simulink model "gm_sampleModel1652_1_sub_sub"  (R2023a)
settings: Solver=VariableStepAuto  StartTime=0.0  StopTime=10.0  RelTol=1e-3
libraries: hdlsllib x7, simulink x2
settings Model: Creator=user1  LastModifiedBy=user1
settings OptimizationCC: BlockReduction=off  ConditionallyExecuteInputs=off
settings DebuggingCC: InheritedTsInSrcMsg=none

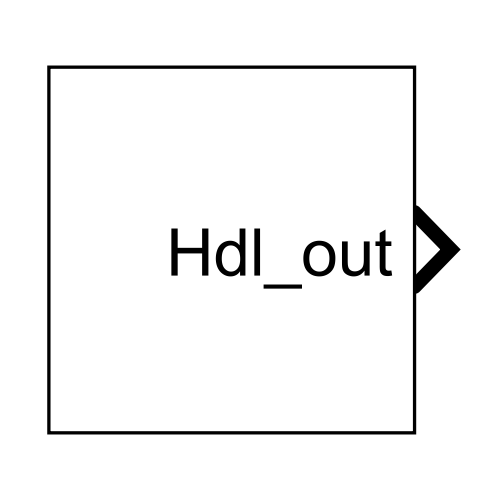
[thumbnail: Simulink's stored preview of the top-level diagram]
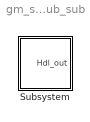
== system gm_sampleModel1652_1_sub_sub ==
  Subsystem : Subsystem

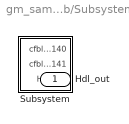
== system gm_sampleModel1652_1_sub_sub/Subsystem ==
  Subsystem : Subsystem
  Hdl_out : Outport  OutDataTypeStr=uint8

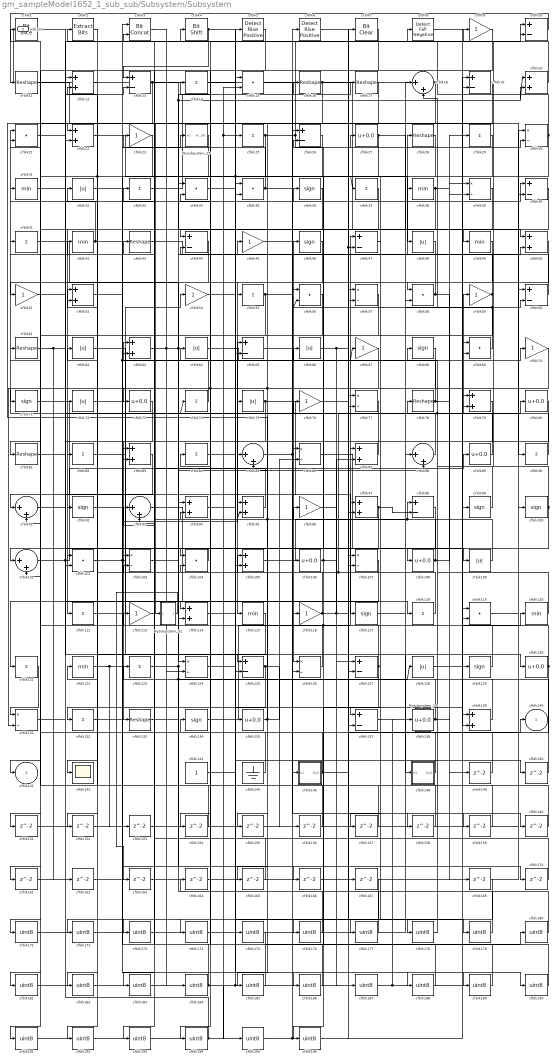
== system gm_sampleModel1652_1_sub_sub/Subsystem/Subsystem ==
  Mysubsystem_15 : Subsystem  TreatAsAtomicUnit=on  RTWFcnName=Mysubsystem_15
      settings: RTWFcnNameOpts=User specified  RTWFileNameOpts=Use function name
  Mysubsystem_19 : Subsystem  TreatAsAtomicUnit=on  RTWFcnName=Mysubsystem_19
      settings: RTWFcnNameOpts=User specified  RTWFileNameOpts=Use function name
  Mysubsystem_31 : Subsystem  TreatAsAtomicUnit=on  RTWFcnName=Mysubsystem_31
      settings: RTWFcnNameOpts=User specified  RTWFileNameOpts=Use function name
  cfblk1 : hdlsllib/Logic and Bit Operations/Bit Slice  lidx=7  ridx=0
  cfblk{10,13,19,26,40,44,47,60,65,98,125,127,137} (13 alike) : Sum  Inputs=+-  OutDataTypeStr=uint8
  cfblk{36,46,68,71,92,99..100,117,129,134} (10 alike) : Signum
  cfblk{18,85,88,91,93,101} (6 alike) : Sum  Inputs=|++  OutDataTypeStr=uint8
  cfblk{15,21,34..35,56,58,69,102,104,119} (10 alike) : DotProduct  OutDataTypeStr=uint8
  cfblk{30,39,57,77,86,103,107,124,126,131} (10 alike) : Product  Inputs=*/  OutDataTypeStr=uint8  RndMeth=Zero  SaturateOnIntegerOverflow=on
  cfblk{12,20,22,50,52,63,79,83,87,94..95,97,105,114,139} (15 alike) : Sum  OutDataTypeStr=uint8
  cfblk{27,73,80,89,106,108,130,135,138} (9 alike) : Bias  Bias=0.0  SaturateOnIntegerOverflow=off
  cfblk{32,48,62,64,66,72,75,109,128} (9 alike) : Abs  OutDataTypeStr=uint8  SaturateOnIntegerOverflow=off
  cfblk{11,16..17,28,43,61,78,81,133} (9 alike) : Reshape
  cfblk{14,25,29,33,37,41,55,74,82,84,90,112,118,121,123,132} (16 alike) : Sum  Inputs=+  OutDataTypeStr=uint8
  cfblk{9,23,45,51,54,59,67,70,76,96,113,116} (12 alike) : Gain  OutDataTypeStr=uint8
  cfblk{31,38,42,49,115,120,122} (7 alike) : MinMax  OutDataTypeStr=uint8
  cfblk142 : Scope
  cfblk144 : Constant  OutDataTypeStr=uint8  SampleTime=-1
  cfblk145 : Ground
  cfblk146 : Subsystem
      settings: LibrarySourceBlock=|
      | hdlsllib/Ports &
      | Subsystems/Subsystem
  cfblk148 : Subsystem
      settings: LibrarySourceBlock=|
      | hdlsllib/Ports &
      | Subsystems/Subsystem
  cfblk{149..167,169..170} (21 alike) : Delay  SampleTime=1
  cfblk{171..196} (26 alike) : DataTypeConversion  OutDataTypeStr=uint8  SaturateOnIntegerOverflow=off  RndMeth=Floor
  cfblk2 : simulink/Logic and Bit Operations/Extract Bits  bitsToExtract=Upper half  numBits=8  bitIdxRange=[0 7]  outScalingMode=Preserve fixed-point scaling
      settings: LibrarySourceBlock=|
      | hdlsllib/Logic and Bit
      | Operations/Extract Bits
  cfblk3 : hdlsllib/Logic and Bit Operations/Bit Concat  numInputs=2
  cfblk4 : hdlsllib/Logic and Bit Operations/Bit Shift  mode=Shift Left Logical  N=0
  cfblk5 : hdlsllib/Logic and Bit Operations/Detect Rise Positive  vinit=0  OutDataTypeStr=uint8
  cfblk6 : hdlsllib/Logic and Bit Operations/Detect Rise Positive  vinit=0  OutDataTypeStr=uint8
  cfblk7 : simulink/Logic and Bit Operations/Bit Clear  iBit=0
      settings: LibrarySourceBlock=|
      | hdlsllib/Logic and Bit
      | Operations/Bit Clear
  cfblk8 : hdlsllib/Logic and Bit Operations/Detect Fall Negative  vinit=0  OutDataTypeStr=uint8
  cfblk140 : Outport  OutDataTypeStr=uint8  VectorParamsAs1DForOutWhenUnconnected=off
  cfblk141 : Outport  Port=2  OutDataTypeStr=uint8  VectorParamsAs1DForOutWhenUnconnected=off
  Hdl_out : Outport  Port=3  OutDataTypeStr=uint8
  wires:
  cfblk125/1 -> cfblk156/1, cfblk132/1
  cfblk106/1 -> cfblk56/1, cfblk127/1
  cfblk67/1 -> cfblk155/1, cfblk131/2
  cfblk130/1 -> cfblk61/1, cfblk134/1
  cfblk72/1 -> cfblk46/1
  cfblk118/1 -> cfblk42/1, cfblk21/1
  cfblk65/1 -> cfblk126/1
  cfblk135/1 -> cfblk86/2, cfblk95/2, cfblk22/1
  cfblk78/1 -> cfblk29/1, cfblk43/1
  cfblk101/1 -> cfblk10/2, cfblk89/1
  cfblk10/1 -> cfblk11/1
  cfblk82/1 -> cfblk54/1
  cfblk99/1 -> cfblk66/1, cfblk74/1
  cfblk18/1 -> Hdl_out/1, cfblk22/2
  cfblk25/1 -> cfblk65/2, cfblk27/1, cfblk10/1
  cfblk59/1 -> cfblk28/1, cfblk56/2, cfblk127/2
  cfblk50/1 -> cfblk115/1
  cfblk29/1 -> cfblk114/1
  cfblk33/1 -> cfblk16/1
  cfblk68/1 -> cfblk112/1
  cfblk90/1 -> cfblk59/1
  cfblk95/1 -> cfblk33/1
  cfblk107/1 -> cfblk121/1
  cfblk93/1 -> cfblk146/1(In1)
  cfblk19/1 -> cfblk181/1
  cfblk40/1 -> cfblk92/1
  cfblk22/1 -> cfblk48/1
  cfblk36/1 -> cfblk44/1
  cfblk47/1 -> cfblk137/1
  cfblk73/1 -> cfblk133/1
  cfblk126/1 -> cfblk52/1
  cfblk108/1 -> cfblk39/2, cfblk65/1
  cfblk146/1(Out1) -> cfblk140/1, cfblk123/1
  cfblk109/1 -> cfblk98/1, cfblk41/1
  cfblk21/1 -> cfblk116/1
  cfblk74/1 -> cfblk63/1
  cfblk89/1 -> cfblk32/1
  cfblk144/1 -> cfblk35/2
  cfblk129/1 -> cfblk62/1
  cfblk62/1 -> cfblk148/1(In1)
  cfblk60/1 -> cfblk14/1
  cfblk134/1 -> cfblk47/1
  cfblk137/1 -> cfblk79/2
  cfblk92/1 -> cfblk108/1
  cfblk4/1 -> cfblk13/1, cfblk37/1, cfblk137/2
  cfblk38/1 -> cfblk161/1, cfblk39/1
  cfblk55/1 -> cfblk73/1, cfblk6/1
  cfblk66/1 -> cfblk167/1, cfblk69/2
  cfblk100/1 -> cfblk177/1, cfblk9/1
  cfblk43/1 -> cfblk45/1
  cfblk30/1 -> cfblk106/1, cfblk2/1
  cfblk16/1 -> cfblk90/1, cfblk125/1
  cfblk71/1 -> cfblk117/1
  cfblk63/1 -> cfblk124/2, cfblk50/2, cfblk118/1
  cfblk51/1 -> cfblk40/1
  cfblk8/1 -> cfblk129/1
  cfblk58/1 -> cfblk169/1, cfblk51/1
  cfblk119/1 -> cfblk100/1
  cfblk105/1 -> cfblk18/1
  cfblk49/1 -> cfblk58/1
  cfblk69/1 -> cfblk18/2
  cfblk112/1 -> cfblk15/1
  cfblk138/1 -> cfblk149/1, cfblk26/2
  cfblk27/1 -> cfblk49/1, cfblk83/2, cfblk105/2
  cfblk86/1 -> cfblk139/1
  cfblk102/1 -> cfblk95/1, cfblk87/1
  cfblk128/1 -> cfblk120/1
  cfblk79/1 -> cfblk83/1
  cfblk120/1 -> cfblk78/1
  cfblk42/1 -> cfblk166/1, cfblk31/1
  cfblk97/1 -> cfblk98/2, cfblk101/1
  cfblk11/1 -> cfblk60/1
  cfblk26/1 -> cfblk71/1
  cfblk1/1 -> cfblk104/1
  cfblk132/1 -> cfblk67/1, Mysubsystem_15/1(In1)
  cfblk2/1 -> cfblk82/1
  cfblk77/1 -> cfblk194/1
  cfblk12/1 -> cfblk102/1
  cfblk87/1 -> cfblk85/1
  cfblk70/1 -> cfblk154/1, cfblk114/2
  cfblk3/1 -> cfblk184/1
  cfblk46/1 -> cfblk91/1
  cfblk104/1 -> cfblk103/1
  cfblk35/1 -> cfblk139/2, cfblk23/1
  cfblk23/1 -> cfblk192/1, cfblk81/1
  cfblk20/1 -> cfblk8/1
  cfblk41/1 -> cfblk124/1
  cfblk75/1 -> cfblk93/2, cfblk107/2
  cfblk64/1 -> cfblk70/1
  cfblk121/1 -> cfblk131/1
  cfblk57/1 -> cfblk191/1
  cfblk13/1 -> cfblk172/1, cfblk50/1
  cfblk80/1 -> cfblk102/2
  cfblk148/1(Out1) -> cfblk122/1
  cfblk44/1 -> cfblk72/1
  cfblk133/1 -> cfblk128/1, cfblk17/1, cfblk20/1
  cfblk81/1 -> cfblk80/1
  cfblk122/1 -> cfblk153/1, cfblk69/1
  cfblk127/1 -> cfblk176/1, cfblk105/1, cfblk76/1
  cfblk131/1 -> cfblk13/2
  cfblk61/1 -> cfblk162/1, cfblk125/2
  cfblk116/1 -> cfblk12/2, cfblk87/2, cfblk30/2, cfblk47/2
  cfblk103/1 -> cfblk88/2
  cfblk85/1 -> cfblk160/1, cfblk38/1
  cfblk31/1 -> cfblk109/1
  cfblk91/1 -> cfblk97/1
  cfblk139/1 -> cfblk4/1
  cfblk54/1 -> cfblk135/1
  cfblk115/1 -> cfblk142/1
  cfblk88/1 -> cfblk75/1
  cfblk56/1 -> cfblk85/2
  cfblk123/1 -> cfblk170/1, cfblk36/1
  cfblk145/1 -> cfblk1/1
  cfblk45/1 -> cfblk130/1
  cfblk96/1 -> cfblk187/1
  cfblk39/1 -> cfblk55/1
  cfblk117/1 -> cfblk60/2
  cfblk114/1 -> cfblk20/2
  cfblk149/1 -> cfblk107/1
  cfblk14/1 -> cfblk150/1
  cfblk150/1 -> cfblk103/2
  cfblk83/1 -> cfblk151/1
  cfblk151/1 -> cfblk79/1
  cfblk48/1 -> cfblk152/1
  cfblk152/1 -> cfblk40/2
  cfblk153/1 -> cfblk119/2
  cfblk154/1 -> cfblk91/2
  cfblk156/1 -> cfblk63/2
  cfblk28/1 -> cfblk157/1
  cfblk157/1 -> cfblk21/2
  cfblk76/1 -> cfblk158/1
  cfblk158/1 -> cfblk52/2
  cfblk15/1 -> cfblk159/1
  cfblk159/1 -> cfblk101/2
  cfblk160/1 -> cfblk104/2
  cfblk161/1 -> cfblk126/2
  cfblk162/1 -> cfblk30/1
  cfblk163/1 -> cfblk88/1
  cfblk164/1 -> cfblk58/2
  cfblk98/1 -> cfblk165/1
  cfblk165/1 -> cfblk44/2
  cfblk166/1 -> cfblk97/2
  cfblk170/1 -> cfblk93/1
  cfblk5/1 -> cfblk171/1
  cfblk171/1 -> cfblk138/1
  cfblk172/1 -> cfblk5/1
  cfblk37/1 -> cfblk173/1
  cfblk173/1 -> cfblk7/1
  cfblk7/1 -> cfblk174/1
  cfblk174/1 -> cfblk64/1
  cfblk94/1 -> cfblk175/1
  cfblk176/1 -> cfblk94/1
  cfblk177/1 -> cfblk94/2
  cfblk34/1 -> cfblk178/1
  cfblk178/1 -> cfblk68/1
  cfblk6/1 -> cfblk179/1
  cfblk179/1 -> cfblk34/1
  cfblk175/1 -> cfblk180/1
  cfblk180/1 -> cfblk34/2
  cfblk181/1 -> cfblk35/1, cfblk26/1
  cfblk167/1 -> cfblk182/1
  cfblk182/1 -> cfblk19/1
  cfblk9/1 -> cfblk183/1
  cfblk183/1 -> cfblk19/2
  cfblk184/1 -> cfblk195/1, cfblk113/1
  cfblk155/1 -> cfblk185/1
  cfblk185/1 -> cfblk3/1
  cfblk32/1 -> cfblk186/1
  cfblk186/1 -> cfblk3/2
  cfblk187/1 -> cfblk119/1, Mysubsystem_19/1(In1)
  cfblk52/1 -> cfblk188/1
  cfblk188/1 -> cfblk96/1
  cfblk84/1 -> cfblk189/1
  cfblk189/1 -> cfblk164/1
  cfblk124/1 -> cfblk190/1
  cfblk190/1 -> cfblk84/1
  cfblk191/1 -> cfblk99/1, cfblk86/1
  cfblk192/1 -> cfblk57/1
  cfblk113/1 -> cfblk193/1
  cfblk193/1 -> cfblk57/2
  cfblk194/1 -> cfblk12/1, cfblk25/1, cfblk15/2
  cfblk195/1 -> cfblk77/1
  cfblk169/1 -> cfblk196/1
  cfblk196/1 -> cfblk77/2
  Mysubsystem_15/1(cfblk141) -> cfblk141/1
  cfblk17/1 -> Mysubsystem_31/1(In1)
  Mysubsystem_31/1(Out1) -> cfblk163/1

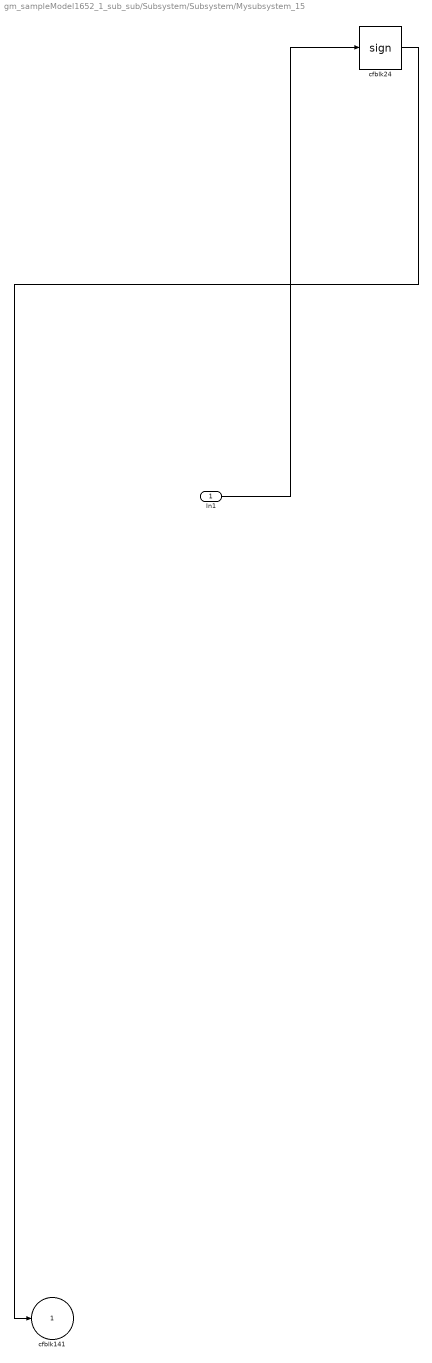
== system gm_sampleModel1652_1_sub_sub/Subsystem/Subsystem/Mysubsystem_15 ==
  In1 : Inport
  cfblk24 : Signum
  cfblk141 : Outport  VectorParamsAs1DForOutWhenUnconnected=off
  wires:
  In1/1 -> cfblk24/1
  cfblk24/1 -> cfblk141/1

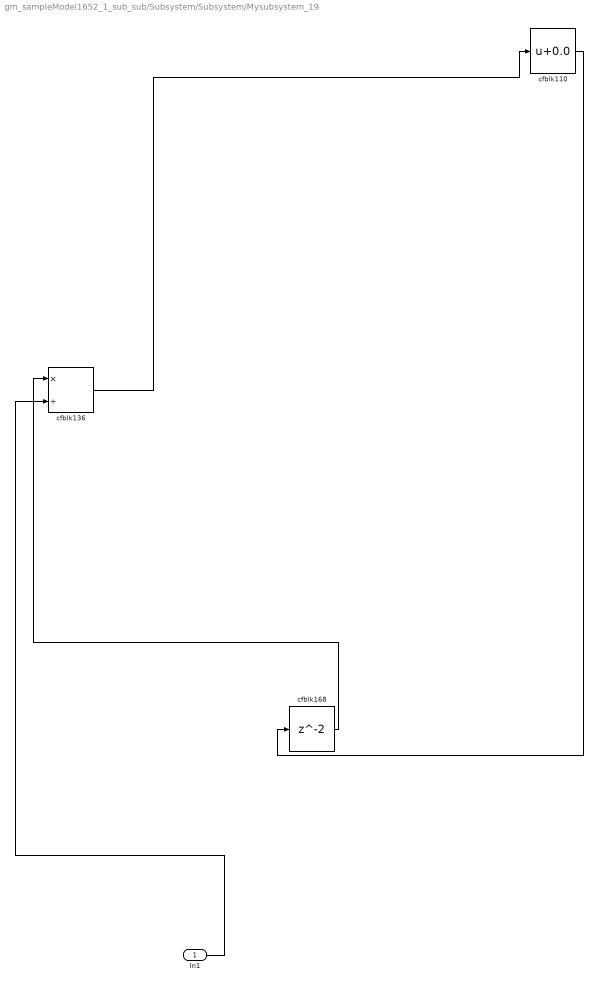
== system gm_sampleModel1652_1_sub_sub/Subsystem/Subsystem/Mysubsystem_19 ==
  In1 : Inport
  cfblk110 : Bias  Bias=0.0  SaturateOnIntegerOverflow=off
  cfblk136 : Product  Inputs=*/  RndMeth=Zero  SaturateOnIntegerOverflow=on
  cfblk168 : Delay  SampleTime=1
  wires:
  In1/1 -> cfblk136/2
  cfblk168/1 -> cfblk136/1
  cfblk110/1 -> cfblk168/1
  cfblk136/1 -> cfblk110/1

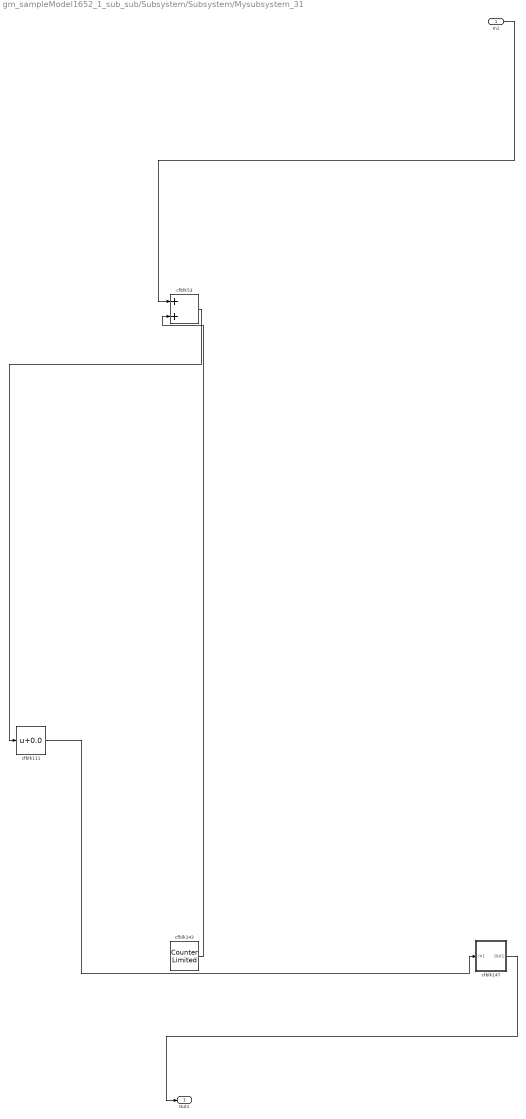
== system gm_sampleModel1652_1_sub_sub/Subsystem/Subsystem/Mysubsystem_31 ==
  In1 : Inport
  cfblk111 : Bias  Bias=0.0  SaturateOnIntegerOverflow=off
  cfblk143 : hdlsllib/Sources/Counter Limited  uplimit=7  tsamp=-1
  cfblk147 : Subsystem
      settings: LibrarySourceBlock=|
      | hdlsllib/Ports &
      | Subsystems/Subsystem
  cfblk53 : Sum
  Out1 : Outport
  wires:
  In1/1 -> cfblk53/1
  cfblk53/1 -> cfblk111/1
  cfblk143/1 -> cfblk53/2
  cfblk147/1(Out1) -> Out1/1
  cfblk111/1 -> cfblk147/1(In1)

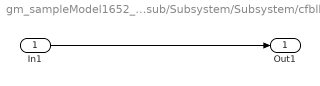
== system gm_sampleModel1652_1_sub_sub/Subsystem/Subsystem/cfblk146 ==
  In1 : Inport
  Out1 : Outport
  wires:
  In1/1 -> Out1/1

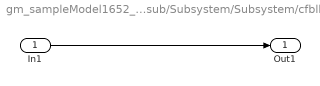
== system gm_sampleModel1652_1_sub_sub/Subsystem/Subsystem/cfblk148 ==
  In1 : Inport
  Out1 : Outport
  wires:
  In1/1 -> Out1/1

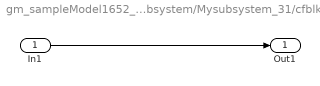
== system gm_sampleModel1652_1_sub_sub/Subsystem/Subsystem/Mysubsystem_31/cfblk147 ==
  In1 : Inport
  Out1 : Outport
  wires:
  In1/1 -> Out1/1
